simulink model "ADC3_IN7_Pot"  (R2013b)
settings: Solver=FixedStepDiscrete  StartTime=0.0  StopTime=10.0  FixedStep=0.1  RelTol=1e-3
undefined symbols (not defined in the file): PC10, PC11, uart4, usart3
libraries: ADC_Lib x3, USART_Lib x2, GPIO_Lib x1
settings Model: Creator=reynaudp  LastModifiedBy=reynaudp
settings OptimizationCC: ExpressionDepthLimit=2147483647  OptimizeModelRefInitCode=on  LifeSpan=1
settings DebuggingCC: StateNameClashWarn=warning
settings HardwareCC: ProdLargestAtomicInteger=Integer  ProdLargestAtomicFloat=Float  ProdIntDivRoundTo=Zero  ProdEndianess=LittleEndian  ProdHWDeviceType=STMicroelectronics->STM32F4xx 32-bit Cortex-M4
settings RTWCC: SystemTargetFile=stm32F4xx.tlc  TemplateMakefile=stm32F4xx.tmf  Description=stm32F4xx (Embedded Target)  GenerateReport=on  ProcessScript=stm32F4xx_make_rtw_hook  IncludeHyperlinkInReport=on  LaunchReport=on
settings CodeAppCC: IgnoreCustomStorageClasses=off  CustomSymbolStrType=$N$R$M  InternalIdentifier=Classic
settings STFCustomTargetCC: ParMdlRefBuildCompliant=on  IncludeMdlTerminateFcn=off  CombineOutputUpdateFcns=on  ERTCustomFileBanners=on  SupportContinuousTime=off  SupportNonInlinedSFcns=off  SupportVariableSizeSignals=on  MATLABClassNameForMDSCustomization=Simulink.SoftwareTarget.ERTCustomization  GRTInterface=off  SystemTargetFile=stm32F4xx.tlc
settings ERTTargetCC: CodeReplacementLibrary=ANSI_C  CompOptLevelCompliant=off  ConcurrentExecutionCompliant=off  IncludeMdlTerminateFcn=off  ERTFirstTimeCompliant=off  SupportVariableSizeSignals=on  ModelStepFunctionPrototypeControlCompliant=off  CPPClassGenCompliant=off  InlinedParameterPlacement=NonHierarchical  ERTSrcFileBannerTemplate=sourceFileTemplate.cgt  ERTHdrFileBannerTemplate=sourceFileTemplate.cgt  ERTDataSrcFileTemplate=sourceFileTemplate.cgt  ERTDataHdrFileTemplate=sourceFileTemplate.cgt  ERTCustomFileTemplate=customRoutineProcess.tlc

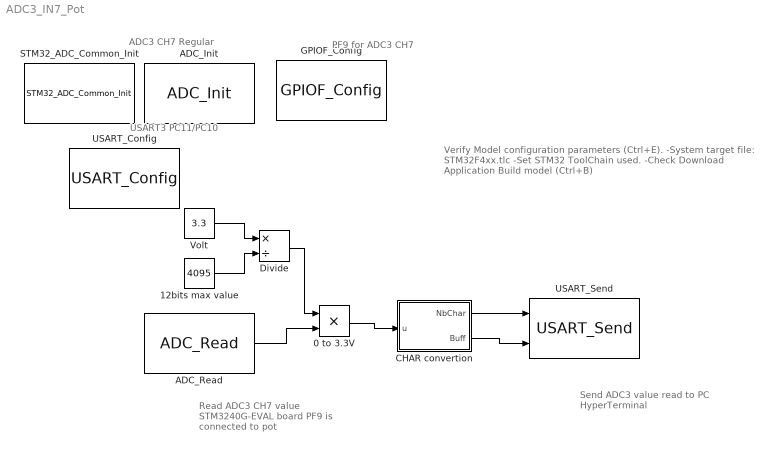
== system ADC3_IN7_Pot ==
  note: Send ADC3 value read to PC
      | HyperTerminal
  note: Read ADC3 CH7 value
      |  STM3240G-EVAL board
      | PF9 is connected to pot
  note: USART3 PC11/PC10
  note: PF9 for ADC3 CH7
  note: ADC3 CH7 Regular
  note: Verify Model configuration parameters (Ctrl+E).
      | 	-System target file: STM32F4xx.tlc
      | 	-Set STM32 ToolChain used.
      | 	-Check Download Application
      | Build model (Ctrl+B)
  0 to 3.3V : Product  RndMeth=Zero
  12bits max value : Constant  Value=4095
  ADC_Init : ADC_Lib/ADC_Init  ADC_Name=ADC3  ADC_Type=Regular  ADC_Default=off  ADC_Offset=0  ADC_Resolution=ADC_Resolution_12b  ADC_ScanConvMode=One_channel  ADC_ContinuousConvMode=on  ADC_ExtTrigPol=ADC_ExternalTrigConvEdge_None  ADC_ExtTrigInjPol=ADC_ExternalTrigInjecConvEdge_None  ADC_ExtTrig=ADC_ExternalTrigConv_T1_CC1  ADC_ExtTrigInj=ADC_ExternalTrigInjecConv_T1_CC4  ADC_DataAlign=ADC_DataAlign_Right  ADC_NbConv=1  ADC_DMA_channel=not_used  ADC_DMA_stream=not_used  ADC_Watchdog_Enable=off  ADC_Watchdog_Command=ADC_AnalogWatchdog_None  ADC_Watchdog_NumChan=0  ADC_Watchdog_HighThreshold=4095  ADC_Watchdog_lowThreshold=0  ADC_Ch0=off  ADC_Ch0T=Regular  ADC_Ch0L=PA0  ADC_Ch1=off  ADC_Ch1T=Regular  ADC_Ch1L=PA1  ADC_Ch2=off  ADC_Ch2T=Regular  ADC_Ch2L=PA2  ADC_Ch3=off  ADC_Ch3T=Regular  ADC_Ch3L=PA3  ADC_Ch4=off  ADC_Ch4T=Regular  ADC_Ch4L=PF6  ADC_Ch5=off  ADC_Ch5T=Regular  ADC_Ch5L=PF7  ADC_Ch6=off  ADC_Ch6T=Regular  ADC_Ch6L=PF8  ADC_Ch7=on  ADC_Ch7T=Regular  ADC_Ch7L=PF9  ADC_Ch8=off  ADC_Ch8T=Regular  ADC_Ch8L=PF10  ADC_Ch9=off  ADC_Ch9T=Regular  ADC_Ch9L=PF3  ADC_Ch10=off  ADC_Ch10T=Regular  ADC_Ch10L=PC0  ADC_Ch11=off  ADC_Ch11T=Regular  ADC_Ch11L=PC1  ADC_Ch12=off  ADC_Ch12T=Regular  ADC_Ch12L=PC2  ADC_Ch13=off  ADC_Ch13T=Regular  ADC_Ch13L=PC3  ADC_Ch14=off  ADC_Ch14T=Regular  ADC_Ch14L=PF4  ADC_Ch15=off  ADC_Ch15T=Regular  ADC_Ch15L=PF5  ADC_Ch16=off  ADC_Ch16T=Regular  ADC_Ch17=off  ADC_Ch17T=Regular  ADC_Ch18=off  ADC_Ch18T=Regular
  ADC_Read : ADC_Lib/ADC_Read  ADC_Name=ADC3  ADC_Ch0=off  ADC_Ch1=off  ADC_Ch2=off  ADC_Ch3=off  ADC_Ch4=off  ADC_Ch5=off  ADC_Ch6=off  ADC_Ch7=on  ADC_Ch8=off  ADC_Ch9=off  ADC_Ch10=off  ADC_Ch11=off  ADC_Ch12=off  ADC_Ch13=off  ADC_Ch14=off  ADC_Ch15=off  ADC_Ch16=off  ADC_Ch17=off  ADC_Ch18=off
  CHAR convertion : MATLAB Function  TreatAsAtomicUnit=on
  Divide : Product  Inputs=*/
  GPIOF_Config : GPIO_Lib/GPIOF_Config  Pin0_Use=off  Pin1_Use=off  Pin2_Use=off  Pin3_Use=off  Pin4_Use=off  Pin5_Use=off  Pin6_Use=off  Pin7_Use=off  Pin8_Use=off  Pin9_Use=on  Pin10_Use=off  Pin11_Use=off  Pin12_Use=off  Pin13_Use=off  Pin14_Use=off  Pin15_Use=off  Pin0_Speed=GPIO_Speed_2MHz  Pin1_Speed=GPIO_Speed_2MHz  Pin2_Speed=GPIO_Speed_2MHz  Pin3_Speed=GPIO_Speed_2MHz  Pin4_Speed=GPIO_Speed_2MHz  Pin5_Speed=GPIO_Speed_2MHz  Pin6_Speed=GPIO_Speed_2MHz  Pin7_Speed=GPIO_Speed_2MHz  Pin8_Speed=GPIO_Speed_2MHz  Pin9_Speed=GPIO_Speed_50MHz  Pin10_Speed=GPIO_Speed_2MHz  Pin11_Speed=GPIO_Speed_2MHz  Pin12_Speed=GPIO_Speed_2MHz  Pin13_Speed=GPIO_Speed_2MHz  Pin14_Speed=GPIO_Speed_2MHz  Pin15_Speed=GPIO_Speed_2MHz  Pin0_Mode=GPIO_Mode_OUT  Pin1_Mode=GPIO_Mode_OUT  Pin2_Mode=GPIO_Mode_OUT  Pin3_Mode=GPIO_Mode_OUT  Pin4_Mode=GPIO_Mode_OUT  Pin5_Mode=GPIO_Mode_OUT  Pin6_Mode=GPIO_Mode_OUT  Pin7_Mode=GPIO_Mode_OUT  Pin8_Mode=GPIO_Mode_OUT  Pin9_Mode=GPIO_Mode_AN  Pin10_Mode=GPIO_Mode_OUT  Pin11_Mode=GPIO_Mode_OUT  Pin12_Mode=GPIO_Mode_OUT  Pin13_Mode=GPIO_Mode_OUT  Pin14_Mode=GPIO_Mode_OUT  Pin15_Mode=GPIO_Mode_OUT  Pin0_Type=GPIO_OType_PP  Pin1_Type=GPIO_OType_PP  Pin2_Type=GPIO_OType_PP  Pin3_Type=GPIO_OType_PP  Pin4_Type=GPIO_OType_PP  Pin5_Type=GPIO_OType_PP  Pin6_Type=GPIO_OType_PP  Pin7_Type=GPIO_OType_PP  Pin8_Type=GPIO_OType_PP  Pin9_Type=GPIO_OType_PP  Pin10_Type=GPIO_OType_PP  Pin11_Type=GPIO_OType_PP  Pin12_Type=GPIO_OType_PP  Pin13_Type=GPIO_OType_PP  Pin14_Type=GPIO_OType_PP  Pin15_Type=GPIO_OType_PP  Pin0_PuPd=GPIO_PuPd_NOPULL  Pin1_PuPd=GPIO_PuPd_NOPULL  Pin2_PuPd=GPIO_PuPd_NOPULL  Pin3_PuPd=GPIO_PuPd_NOPULL  Pin4_PuPd=GPIO_PuPd_NOPULL  Pin5_PuPd=GPIO_PuPd_NOPULL  Pin6_PuPd=GPIO_PuPd_NOPULL  Pin7_PuPd=GPIO_PuPd_NOPULL  Pin8_PuPd=GPIO_PuPd_NOPULL  Pin9_PuPd=GPIO_PuPd_NOPULL  Pin10_PuPd=GPIO_PuPd_NOPULL  Pin11_PuPd=GPIO_PuPd_NOPULL  Pin12_PuPd=GPIO_PuPd_NOPULL  Pin13_PuPd=GPIO_PuPd_NOPULL  Pin14_PuPd=GPIO_PuPd_NOPULL  Pin15_PuPd=GPIO_PuPd_NOPULL  Pin0_AF=GPIO_AF_I2C2  Pin1_AF=GPIO_AF_FSMC  Pin2_AF=GPIO_AF_I2C2  Pin3_AF=GPIO_AF_FSMC  Pin4_AF=GPIO_AF_FSMC  Pin5_AF=GPIO_AF_EVENTOUT  Pin6_AF=GPIO_AF_TIM10  Pin7_AF=GPIO_AF_TIM11  Pin8_AF=GPIO_AF_TIM13  Pin9_AF=GPIO_AF_TIM14  Pin10_AF=GPIO_AF_FSMC  Pin11_AF=GPIO_AF_DCMI  Pin12_AF=GPIO_AF_FSMC  Pin13_AF=GPIO_AF_FSMC  Pin14_AF=GPIO_AF_FSMC  Pin15_AF=GPIO_AF_EVENTOUT  Pin0_Set=off  Pin1_Set=off  Pin2_Set=off  Pin3_Set=off  Pin4_Set=off  Pin5_Set=off  Pin6_Set=off  Pin7_Set=off  Pin8_Set=off  Pin9_Set=off  Pin10_Set=off  Pin11_Set=off  Pin12_Set=off  Pin13_Set=off  Pin14_Set=off  Pin15_Set=off
  STM32_ADC_Common_Init : ADC_Lib/STM32_ADC_Common_Init  ADC_Mode=ADC_Mode_Independent  ADC_Prescaler=ADC_Prescaler_Div2  ADC_DMAAccessMode=ADC_DMAAccessMode_Disabled  ADC_TwoSamplingDelay=ADC_TwoSamplingDelay_5Cycles
  USART_Config : USART_Lib/USART_Config  USART_CONFIG=USART3  USART_CONFIG_PIN=PC11/PC10 : (usart3 / uart4)  USART_SPEED=115200  USART_DATA=USART_WordLength_8b  USART_PARITY=USART_Parity_No  USART_STOP=USART_StopBits_1  USART_FLOW=on  USART_DEFAULT=off  It_rcv=off  It_send=on  Def_handler=on  Cust_handler=USART3_IRQHandler
  USART_Send : USART_Lib/USART_Send  USART_name=USART3  USART_buff=20
  Volt : Constant  Value=3.3  OutDataTypeStr=single
  wires:
  Volt/1 -> Divide/1
  12bits max value/1 -> Divide/2
  Divide/1 -> 0 to 3.3V/1
  ADC_Read/1 -> 0 to 3.3V/2
  0 to 3.3V/1 -> CHAR convertion/1(u)
  CHAR convertion/2(Buff) -> USART_Send/2
  CHAR convertion/1(NbChar) -> USART_Send/1

== matlab function ADC3_IN7_Pot/CHAR convertion ==
  data: u input; NbChar output uint16 size=1; Buff output uint8 size=[1 20]
function [NbChar, Buff] = convert(u)
%%Buff = uint32(0);
buffer = zeros(1,15,'uint8');
strLen = int32(0);
strLen = coder.ceval('sprintf',coder.wref(buffer),['%2.2f',0],u);
%tmp = buffer(1:strLen);
tmp = uint8('Volt');
y= [buffer(1:4), tmp, 13, 10, 0];
%%Buff = uint32(coder.ref(y));
Buff = [buffer(1:4), tmp, 13, 10, 0];
NbChar = uint16(size(y,2));
